simulink model "TPS_SWC_test"  (R2022b)
settings: Solver=VariableStepAuto  StartTime=0.0  StopTime=2  RelTol=1e-3
undefined symbols (not defined in the file or in its folder): sigbuilder_block
settings Model: Creator=yasso  LastModifiedBy=yasso

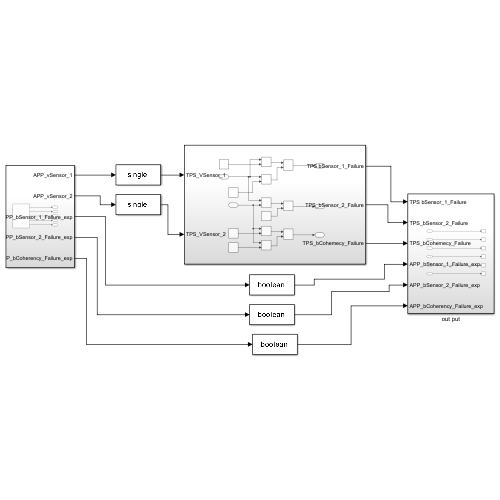
[thumbnail: Simulink's stored preview of the top-level diagram]
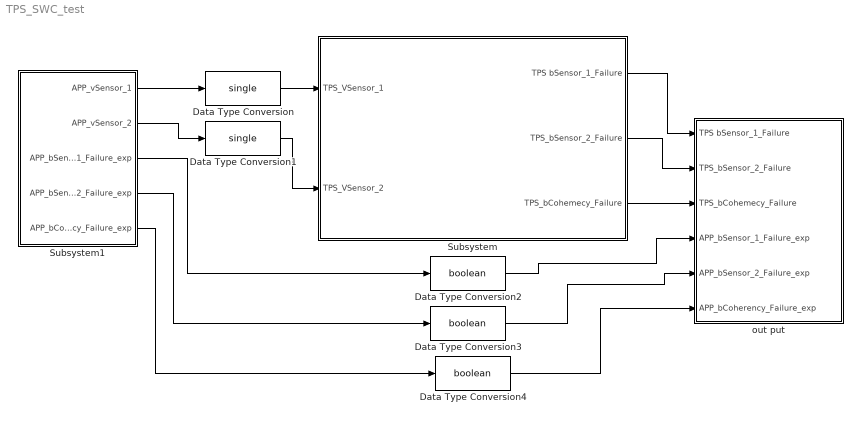
== system TPS_SWC_test ==
  Data Type Conversion : DataTypeConversion  OutDataTypeStr=single  SaturateOnIntegerOverflow=off  RndMeth=Floor
  Data Type Conversion1 : DataTypeConversion  OutDataTypeStr=single  SaturateOnIntegerOverflow=off  RndMeth=Floor
  Data Type Conversion2 : DataTypeConversion  OutDataTypeStr=boolean  SaturateOnIntegerOverflow=off  RndMeth=Floor
  Data Type Conversion3 : DataTypeConversion  OutDataTypeStr=boolean  SaturateOnIntegerOverflow=off  RndMeth=Floor
  Data Type Conversion4 : DataTypeConversion  OutDataTypeStr=boolean  SaturateOnIntegerOverflow=off  RndMeth=Floor
  Subsystem : Subsystem
  Subsystem1 : Subsystem
  out put : Subsystem
  wires:
  Subsystem1/5(APP_bCoherency_Failure_exp) -> Data Type Conversion4/1
  Subsystem1/4(APP_bSensor_2_Failure_exp) -> Data Type Conversion3/1
  Subsystem1/3(APP_bSensor_1_Failure_exp) -> Data Type Conversion2/1
  Subsystem1/2(APP_vSensor_2) -> Data Type Conversion1/1
  Subsystem1/1(APP_vSensor_1) -> Data Type Conversion/1
  Data Type Conversion/1 -> Subsystem/1(TPS_VSensor_1)
  Data Type Conversion1/1 -> Subsystem/2(TPS_VSensor_2)
  Data Type Conversion4/1 -> out put/6(APP_bCoherency_Failure_exp)
  Subsystem/1(TPS bSensor_1_Failure) -> out put/1(TPS bSensor_1_Failure)
  Subsystem/2(TPS_bSensor_2_Failure) -> out put/2(TPS_bSensor_2_Failure)
  Subsystem/3(TPS_bCohemecy_Failure) -> out put/3(TPS_bCohemecy_Failure)
  Data Type Conversion2/1 -> out put/4(APP_bSensor_1_Failure_exp)
  Data Type Conversion3/1 -> out put/5(APP_bSensor_2_Failure_exp)

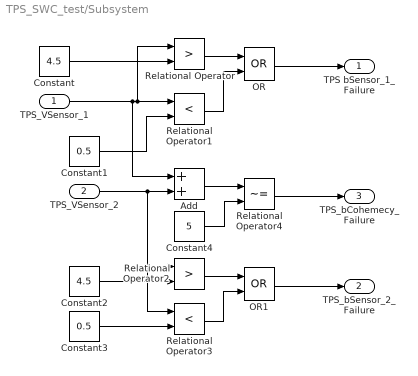
== system TPS_SWC_test/Subsystem ==
  TPS_VSensor_1 : Inport  OutDataTypeStr=single
  TPS_VSensor_2 : Inport  Port=2  OutDataTypeStr=single
  Add : Sum
  Constant : Constant  Value=4.5
  Constant1 : Constant  Value=0.5
  Constant2 : Constant  Value=4.5
  Constant3 : Constant  Value=0.5
  Constant4 : Constant  Value=5
  OR : Logic  Operator=OR  AllPortsSameDT=off  OutDataTypeStr=boolean
  OR1 : Logic  Operator=OR  AllPortsSameDT=off  OutDataTypeStr=boolean
  Relational Operator : RelationalOperator  Operator=>  OutDataTypeStr=boolean  RndMeth=Simplest  InputSameDT=off
  Relational Operator1 : RelationalOperator  Operator=<  OutDataTypeStr=boolean  RndMeth=Simplest  InputSameDT=off
  Relational Operator2 : RelationalOperator  Operator=>  OutDataTypeStr=boolean  RndMeth=Simplest  InputSameDT=off
  Relational Operator3 : RelationalOperator  Operator=<  OutDataTypeStr=boolean  RndMeth=Simplest  InputSameDT=off
  Relational Operator4 : RelationalOperator  Operator=~=  OutDataTypeStr=boolean  RndMeth=Simplest  InputSameDT=off
  TPS bSensor_1_Failure : Outport  OutDataTypeStr=boolean
  TPS_bSensor_2_Failure : Outport  Port=2  OutDataTypeStr=boolean
  TPS_bCohemecy_Failure : Outport  Port=3  OutDataTypeStr=boolean
  wires:
  Relational Operator1/1 -> OR/2
  Relational Operator/1 -> OR/1
  Constant/1 -> Relational Operator/2
  Constant1/1 -> Relational Operator1/2
  TPS_VSensor_1/1 -> Relational Operator/1, Relational Operator1/1, Add/1
  TPS_VSensor_2/1 -> Relational Operator3/1, Relational Operator2/1, Add/2
  Constant3/1 -> Relational Operator3/2
  Constant2/1 -> Relational Operator2/2
  Add/1 -> Relational Operator4/1
  Constant4/1 -> Relational Operator4/2
  Relational Operator2/1 -> OR1/1
  Relational Operator3/1 -> OR1/2
  OR/1 -> TPS bSensor_1_Failure/1
  Relational Operator4/1 -> TPS_bCohemecy_Failure/1
  OR1/1 -> TPS_bSensor_2_Failure/1

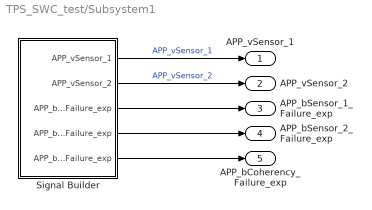
== system TPS_SWC_test/Subsystem1 ==
  Signal Builder : Subsystem  Tag=STV Subsys  LoadFcn=sigbuilder_block('load');  StartFcn=sigbuilder_block('start');  StopFcn=sigbuilder_block('stop');  ClipboardFcn=sigbuilder_block('clipboard');  mask(Sigbuilder block){tuvar=[0:10]}
      mask help: Simulink:masks:SigbuilderBlock_MD
      mask init:
      | if ~strcmp(get_param(bdroot(gcbh),'SimulationStatus'),'stopped') tuvar = sigbuilder_block('maskInit'); end
      settings: CopyFcn=sigbuilder_block('copy');  DeleteFcn=sigbuilder_block('delete');  ModelCloseFcn=sigbuilder_block('modelClose');  PreSaveFcn=sigbuilder_block('preSave');  PauseFcn=sigbuilder_block('pause');  ContinueFcn=sigbuilder_block('continue');  NameChangeFcn=sigbuilder_block('namechange');  OpenFcn=sigbuilder_block('open',[430.2 110.4 550.8 400.2 ]);  CloseFcn=sigbuilder_block('close');
      mask Display: plot(0, 0, 100, 100,[2, 2, 32, 32, 2], [68, 8, 8, 68, 68],[32, 2], [38, 38], [32, 19, 2],[53, 60, 44], [32, 17, 17, 2],[16, 16, 31, 31]);txt = getActiveGroup(gcbh);text(2, 100, txt,'verticalAlignment', 'top');
  APP_vSensor_1 : Outport
  APP_vSensor_2 : Outport  Port=2
  APP_bSensor_1_Failure_exp : Outport  Port=3
  APP_bSensor_2_Failure_exp : Outport  Port=4
  APP_bCoherency_Failure_exp : Outport  Port=5
  wires:
  Signal Builder/1(APP_vSensor_1) -> APP_vSensor_1/1  "APP_vSensor_1"
  Signal Builder/4(APP_bSensor_2_Failure_exp) -> APP_bSensor_2_Failure_exp/1
  Signal Builder/2(APP_vSensor_2) -> APP_vSensor_2/1  "APP_vSensor_2"
  Signal Builder/5(APP_bCoherency_Failure_exp) -> APP_bCoherency_Failure_exp/1
  Signal Builder/3(APP_bSensor_1_Failure_exp) -> APP_bSensor_1_Failure_exp/1

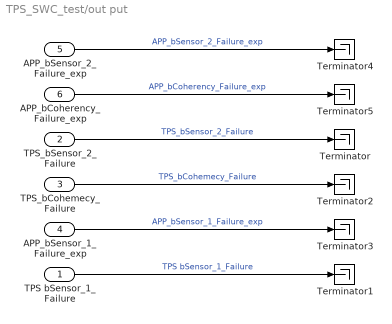
== system TPS_SWC_test/out put ==
  TPS bSensor_1_Failure : Inport
  TPS_bSensor_2_Failure : Inport  Port=2
  TPS_bCohemecy_Failure : Inport  Port=3
  APP_bSensor_1_Failure_exp : Inport  Port=4
  APP_bSensor_2_Failure_exp : Inport  Port=5
  APP_bCoherency_Failure_exp : Inport  Port=6
  Terminator{,1..5} (6 alike) : Terminator
  wires:
  APP_bSensor_1_Failure_exp/1 -> Terminator3/1  "APP_bSensor_1_Failure_exp"
  APP_bSensor_2_Failure_exp/1 -> Terminator4/1  "APP_bSensor_2_Failure_exp"
  TPS bSensor_1_Failure/1 -> Terminator1/1  "TPS bSensor_1_Failure"
  TPS_bCohemecy_Failure/1 -> Terminator2/1  "TPS_bCohemecy_Failure"
  TPS_bSensor_2_Failure/1 -> Terminator/1  "TPS_bSensor_2_Failure"
  APP_bCoherency_Failure_exp/1 -> Terminator5/1  "APP_bCoherency_Failure_exp"

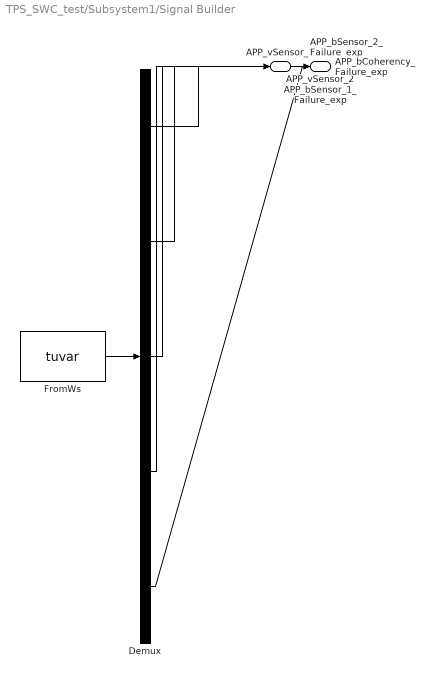
== system TPS_SWC_test/Subsystem1/Signal Builder ==
  Demux : Demux  Tag=STV Demux  Outputs=5
      settings: DisplayOption=none
  FromWs : FromWorkspace  Tag=STV FromWs  VariableName=tuvar
      SigBuilderData=|
      | common.afterFinalStr = 'Extrapolate'
      | common.sampleTime = 0
      | dataSet.timeRange = [0 2]
      | dataSet.name = 'Sheet1'
      | sbobj.Name = 'Signal Builder'
      | sbobj.Groups.Name = 'Sheet1'
      | sbobj.Groups.Signals(1).Name = 'APP_vSensor_1'
      | sbobj.Groups.Signals(1).XData = [0 1 2]
      | sbobj.Groups.Signals(1).YData = [0.5 4.5 0.5]
      | sbobj.Groups.Signals(2).Name = 'APP_vSensor_2'
      | sbobj.Groups.Signals(2).XData = [0 1 2]
      | sbobj.Groups.Signals(2).YData = [4.5 0.5 4.5]
      | sbobj.Groups.Signals(3).Name = 'APP_bSensor_1_Failure_exp'
      | sbobj.Groups.Signals(3).XData = [0 1 2]
      | sbobj.Groups.Signals(3).YData = [0 0 0]
      | sbobj.Groups.Signals(4).Name = 'APP_bSensor_2_Failure_exp'
      | sbobj.Groups.Signals(4).XData = [0 1 2]
      | sbobj.Groups.Signals(4).YData = [0 0 0]
      | sbobj.Groups.Signals(5).Name = 'APP_bCoherency_Failure_exp'
      | sbobj.Groups.Signals(5).XData = [0 1 2]
      | sbobj.Groups.Signals(5).YData = [0 0 0]
      | sbobj.Groups.TimeRange = [0 2]
  APP_vSensor_1 : Outport  Tag=STV Outport
  APP_vSensor_2 : Outport  Tag=STV Outport  Port=2
  APP_bSensor_1_Failure_exp : Outport  Tag=STV Outport  Port=3
  APP_bSensor_2_Failure_exp : Outport  Tag=STV Outport  Port=4
  APP_bCoherency_Failure_exp : Outport  Tag=STV Outport  Port=5
  wires:
  Demux/1 -> APP_vSensor_1/1
  FromWs/1 -> Demux/1
  Demux/2 -> APP_vSensor_2/1
  Demux/3 -> APP_bSensor_1_Failure_exp/1
  Demux/4 -> APP_bSensor_2_Failure_exp/1
  Demux/5 -> APP_bCoherency_Failure_exp/1
